simulink model "test_fmu_step_input"  (R2022a)
settings: Solver=VariableStepAuto  StartTime=0.0  StopTime=10.0  RelTol=1e-3
settings Model: Creator=lordx  LastModifiedBy=lordx

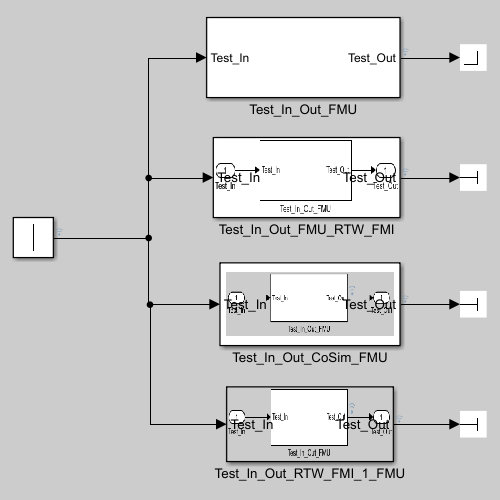
[thumbnail: Simulink's stored preview of the top-level diagram]
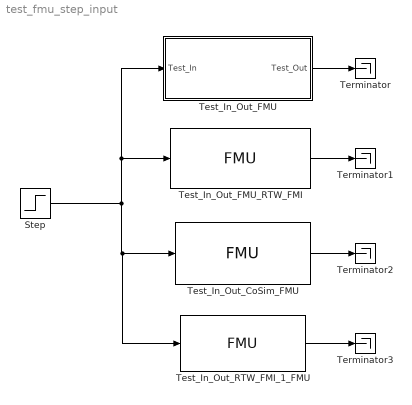
== system test_fmu_step_input ==
  Step : Step  SampleTime=0
  Terminator{,1..3} (4 alike) : Terminator
  Test_In_Out_CoSim_FMU : FMU  FMUName=test_fmu_v1.fmu  FMUDebugLogging=on  FMUMode=CoSimulation  FMUIsToleranceUsed=on  FMUCreateBusObject=off
      mask Type: test_fmu_v1 [Co-Simulation, v2.0]
      mask Display:
      | if (exist([Simulink.fileGenControl('get','CacheFolder') '\slprj\_fmu\df234959f4d02ba7b2a74bdaf3376e61\test_fmu_v1\model.png'],'file'))
      |     image([Simulink.fileGenControl('get','CacheFolder') '\slprj\_fmu\df234959f4d02ba7b2a74bdaf3376e61\test_fmu_v1\model.png']);
      | else
      |     disp('test_fmu_v1');
      | end
      | port_label('output',1,'Test_Out');
      | port_label('input',1,'Test_In');
  Test_In_Out_FMU : Subsystem
  Test_In_Out_FMU_RTW_FMI : FMU  FMUName=test_fmu.fmu  FMUDebugLogging=on  FMUMode=CoSimulation  Parameters_Gain_Gain=10  mask(test_fmu [Co-Simulation, v3.0]){}
      mask Display:
      | if (exist([Simulink.fileGenControl('get','CacheFolder') '\slprj\_fmu\5bc003257c4629cc1c641c27e917a90f\test_fmu\model.png'],'file'))
      |     image([Simulink.fileGenControl('get','CacheFolder') '\slprj\_fmu\5bc003257c4629cc1c641c27e917a90f\test_fmu\model.png']);
      | else
      |     disp('test_fmu [Co-Simulation, v3.0]');
      | end
      | port_label('output',1,'Test_Out');
      | port_label('input',1,'Test_In');
  Test_In_Out_RTW_FMI_1_FMU : FMU  FMUName=test_fmu_v2.fmu  FMUDebugLogging=on  FMUMode=CoSimulation
      mask Type: test_fmu_v2 [Co-Simulation, v3.0]
      mask Display:
      | if (exist([Simulink.fileGenControl('get','CacheFolder') '\slprj\_fmu\0c353e60cd310a1482f165b4d2a72862\test_fmu_v2\model.png'],'file'))
      |     image([Simulink.fileGenControl('get','CacheFolder') '\slprj\_fmu\0c353e60cd310a1482f165b4d2a72862\test_fmu_v2\model.png']);
      | else
      |     disp('test_fmu_v2 [Co-Simulation, v3.0]');
      | end
      | port_label('output',1,'Test_Out');
      | port_label('input',1,'Test_In');
  wires:
  Step/1 -> Test_In_Out_RTW_FMI_1_FMU/1, Test_In_Out_CoSim_FMU/1, Test_In_Out_FMU/1(Test_In), Test_In_Out_FMU_RTW_FMI/1
  Test_In_Out_FMU_RTW_FMI/1 -> Terminator1/1
  Test_In_Out_FMU/1(Test_Out) -> Terminator/1
  Test_In_Out_CoSim_FMU/1 -> Terminator2/1
  Test_In_Out_RTW_FMI_1_FMU/1 -> Terminator3/1

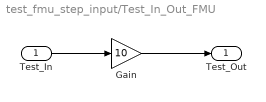
== system test_fmu_step_input/Test_In_Out_FMU ==
  Test_In : Inport
  Gain : Gain  Gain=10
  Test_Out : Outport
  wires:
  Test_In/1 -> Gain/1
  Gain/1 -> Test_Out/1
